simulink model "vehicle_dynamics"  (R2015a)
settings: Solver=ode45  StartTime=0.0  StopTime=10.0  RelTol=1e-3
undefined symbols (not defined in the file): h, I_z, J_wfl, J_wfr, J_wrl, J_wrr, l, l_f, l_r, l_w, m
settings Model: Creator=BML  LastModifiedBy=BML

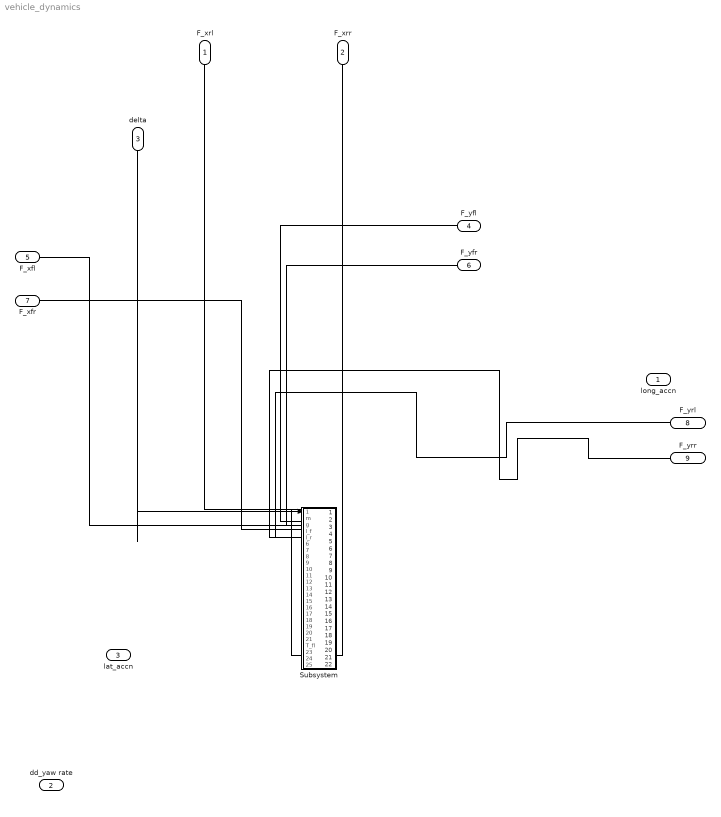
== system vehicle_dynamics ==
  F_xrl : Inport
  F_xrr : Inport  Port=2
  delta : Inport  Port=3
  F_yfl : Inport  Port=4
  F_xfl : Inport  Port=5
  F_yfr : Inport  Port=6
  F_xfr : Inport  Port=7
  F_yrl : Inport  Port=8
  F_yrr : Inport  Port=9
  Subsystem : Subsystem
  long_accn : Outport
  dd_yaw rate : Outport  Port=2
  lat_accn : Outport  Port=3
  wires:
  F_xrl/1 -> ?
  F_xrr/1 -> ?
  delta/1 -> Subsystem/1(delta)
  F_yfl/1 -> ?
  F_xfl/1 -> ?
  F_yfr/1 -> ?
  F_xfr/1 -> ?
  F_yrl/1 -> ?
  F_yrr/1 -> ?
  ? -> long_accn/1
  ? -> dd_yaw rate/1
  ? -> lat_accn/1

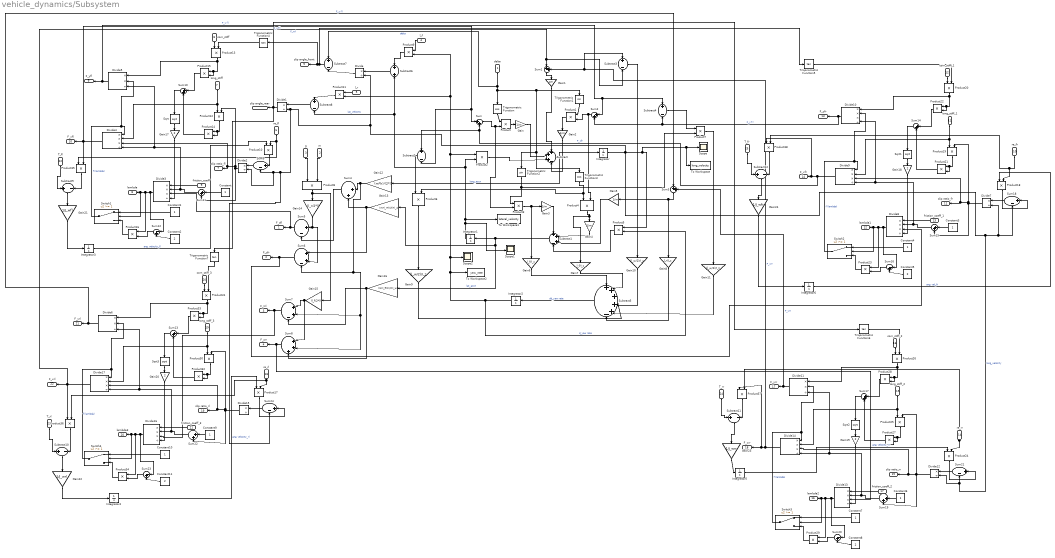
== system vehicle_dynamics/Subsystem ==
  delta : Inport
  m : Inport  Port=2
  g : Inport  Port=3
  l_f : Inport  Port=4
  l_r : Inport  Port=5
  "re_fl " : Inport  Port=6
  "Iong_stiff " : Inport  Port=7
  corn_stiff : Inport  Port=8
  friction_coeff : Inport  Port=9
  "re_fr " : Inport  Port=10
  Iong_stiff_1 : Inport  Port=11
  "corn_stiff_1 " : Inport  Port=12
  friction_coeff_1 : Inport  Port=13
  "re_rr " : Inport  Port=14
  Iong_stiff_2 : Inport  Port=15
  corn_stiff_2 : Inport  Port=16
  friction_coeff_2 : Inport  Port=17
  re_rl : Inport  Port=18
  Iong_stiff_3 : Inport  Port=19
  corn_stiff_3 : Inport  Port=20
  "      friction_coeff_3" : Inport  Port=21
  T_fl : Inport  Port=22
  "T_rl " : Inport  Port=23
  "T_rr " : Inport  Port=24
  "T_fr " : Inport  Port=25
  Constant{,1,3..4,6..7,9..10} (8 alike) : Constant
  Constant{2,5,8,11} (4 alike) : Constant  Value=2
  Divide{,1..2,7,12,15} (6 alike) : Product  Inputs=*/
  Divide{3..4,8..10,13..14,16..17} (9 alike) : Product  Inputs=***/
  Divide11 : Product  Inputs=**/
  Divide5 : Product  Inputs=**/
  Divide6 : Product  Inputs=**/
  Gain{,1..5} (6 alike) : Gain  Gain=1/m
  Gain10 : Gain  Gain=(l_w/2)/I_z
  Gain11 : Gain  Gain=(l_w/2)/I_z
  Gain12 : Gain  Gain=(m*h)/(2*l)
  Gain13 : Gain  Gain=(m*l_r*h)/(l*l_w)
  Gain14 : Gain  Gain=(l_r/2*l)
  Gain15 : Gain  Gain=(l_f/2*l)
  Gain16 : Gain  Gain=(m*l_f*h)/(l*l_w)
  Gain{17..20} (4 alike) : Gain  Gain=2
  Gain21 : Gain  Gain=1/J_wfl
  Gain22 : Gain  Gain=1/J_wrl
  Gain23 : Gain  Gain=1/J_wrr
  Gain24 : Gain  Gain=1/J_wfr
  Gain6 : Gain  Gain=l_f/I_z
  Gain7 : Gain  Gain=l_f/I_z
  Gain8 : Gain  Gain=l_r/I_z
  Gain9 : Gain  Gain=(l_w/2)/I_z
  Integrator{,1..6} (7 alike) : Integrator
  Product{,1..38} (39 alike) : Product
  Scope : Scope
  Scope1 : Scope
  Scope2 : Scope
      settings: SaveName=ScopeData2
  Sqrt{,1..3} (4 alike) : Sqrt  SaturateOnIntegerOverflow=on
  Subtract : Sum  Inputs=+++-
  Subtract1 : Sum  Inputs=+++-
  Subtract{2..4,7..12} (9 alike) : Sum  Inputs=+-
  Subtract5 : Sum  Inputs=+++++-
  Subtract6 : Sum
  Sum{,1..4,10..11,13..15,17,19,22} (13 alike) : Sum  Inputs=|++
  Sum{12,16,20,23} (4 alike) : Sum  Inputs=|-+
  Sum{5,9,18,21,24} (5 alike) : Sum  Inputs=|+-
  Sum6 : Sum  Inputs=|++-
  Sum7 : Sum  Inputs=|++-
  Sum8 : Sum  Inputs=|+++
  Switch{1..4} (4 alike) : Switch  Threshold=1
  To Workspace : ToWorkspace  VariableName=long_velocity  SaveFormat=Timeseries  SampleTime=-1
  To Workspace1 : ToWorkspace  VariableName=lateral_velocity  SaveFormat=Timeseries  SampleTime=-1
  To Workspace2 : ToWorkspace  VariableName=yaw_rate  SaveFormat=Timeseries  SampleTime=-1
  Trigonometric Function : Trigonometry  Operator=cos
  Trigonometric Function1 : Trigonometry
  Trigonometric Function2 : Trigonometry
  Trigonometric Function3 : Trigonometry  Operator=cos
  Trigonometric Function{4..7} (4 alike) : Trigonometry  Operator=tan
  F_zfl : Outport
  F_zfr : Outport  Port=2
  F_zrl : Outport  Port=3
  F_zrr : Outport  Port=4
  slip angle_front : Outport  Port=5
  slip angle_rear : Outport  Port=6
  slip ratio_fl : Outport  Port=7
  lambda : Outport  Port=8
  "F_yfl " : Outport  Port=9
  "F_xfl " : Outport  Port=10
  slip ratio_fr : Outport  Port=11
  lambda1 : Outport  Port=12
  F_yfr : Outport  Port=13
  F_xfr : Outport  Port=14
  slip ratio_rr : Outport  Port=15
  lambda2 : Outport  Port=16
  F_yrr : Outport  Port=17
  F_xrr : Outport  Port=18
  slip ratio_rl : Outport  Port=19
  lambda3 : Outport  Port=20
  F_yrl : Outport  Port=21
  "F_xrl " : Outport  Port=22
  wires:
  Gain10/1 -> Subtract5/4
  Product2/1 -> Subtract/3
  Gain11/1 -> Subtract5/5
  Sum3/1 -> Gain5/1, Gain8/1
  Integrator1/1 -> Scope1/1, Subtract8/2, Subtract6/2, Product2/2, To Workspace1/1  "lat_velocity"
  Subtract3/1 -> Gain10/1
  Gain3/1 -> Subtract1/1
  Product5/1 -> Subtract1/4
  Integrator2/1 -> Product5/2, To Workspace2/1, Scope2/1, Product9/2, Product11/2, Product2/1  "d_yaw rate"
  Trigonometric Function3/1 -> Product6/2, Product4/1
  Product7/1 -> Gain11/1
  Product4/1 -> Gain7/1, Gain4/1
  Trigonometric Function1/1 -> Product1/1
  Gain4/1 -> Subtract1/2
  Product3/1 -> Gain6/1, Gain3/1
  Subtract4/1 -> Product7/1
  Gain/1 -> Subtract/2
  Trigonometric Function/1 -> Product/1
  Sum/1 -> Product3/2, Product/2
  Product/1 -> Gain/1
  Subtract/1 -> Integrator/1, Gain12/1  "long_accn"
  Gain6/1 -> Subtract5/1
  Gain5/1 -> Subtract1/3
  Sum1/1 -> Gain1/1
  Subtract1/1 -> Integrator1/1, Gain13/1, Gain16/1  "lat_accn"
  Gain2/1 -> Subtract/4
  Product1/1 -> Gain2/1
  Trigonometric Function2/1 -> Product3/1, Product7/2
  Sum2/1 -> Product1/2, Product4/2
  Gain8/1 -> Subtract5/6
  Gain7/1 -> Subtract5/2
  Product6/1 -> Gain9/1
  Gain9/1 -> Subtract5/3
  Subtract5/1 -> Integrator2/1  "dd_yaw rate"
  Gain1/1 -> Subtract/1
  Subtract2/1 -> Product6/1
  Gain13/1 -> Sum4/2, Sum6/1
  g/1 -> Product8/1
  m/1 -> Product8/2
  Sum5/1 -> Divide3/3, F_zfl/1
  Gain14/1 -> Sum6/2, Sum5/1
  Product8/1 -> Gain15/1, Gain14/1
  Gain12/1 -> Sum8/2, Sum7/2, Sum6/3, Sum4/1
  Gain15/1 -> Sum8/1, Sum7/1
  Sum4/1 -> Sum5/2
  Gain16/1 -> Sum8/3, Sum7/3
  l_f/1 -> Product9/1
  Product9/1 -> Subtract6/1
  Subtract6/1 -> Divide/1
  delta/1 -> Subtract7/1, Trigonometric Function/1, Trigonometric Function3/1, Trigonometric Function2/1, Trigonometric Function1/1  "delta"
  l_r/1 -> Product11/1
  Product11/1 -> Subtract8/1
  Divide/1 -> Subtract7/2
  Subtract8/1 -> Divide1/1
  Product10/1 -> Sum9/1
  Sum9/1 -> Divide2/1
  "Iong_stiff "/1 -> Divide4/2, Product12/1
  Divide2/1 -> Product12/2, Divide4/3, slip ratio_fl/1, Sum11/2
  corn_stiff/1 -> Product13/1
  Subtract7/1 -> Trigonometric Function5/1, Trigonometric Function4/1, slip angle_front/1
  Product12/1 -> Product14/2, Product14/1
  Trigonometric Function4/1 -> Product13/2
  Product13/1 -> Product15/2, Product15/1, Divide5/1
  Product14/1 -> Sum10/2
  Product15/1 -> Sum10/1
  Sum10/1 -> Sqrt/1
  Sqrt/1 -> Gain17/1
  Constant/1 -> Sum11/1
  Gain17/1 -> Divide3/4
  friction_coeff/1 -> Divide3/1
  Sum11/1 -> Divide5/3, Divide4/4, Divide3/2
  Divide3/1 -> Product16/1, Switch1/2, lambda/1, Sum12/1
  Constant1/1 -> Switch1/1
  Constant2/1 -> Sum12/2
  Sum12/1 -> Product16/2
  Product16/1 -> Switch1/3
  Switch1/1 -> Divide5/2, Divide4/1  "f (lambda)"
  Divide4/1 -> Sum/1, Subtract2/2, "F_xfl "/1, Product35/2  "F_x f l"
  Integrator/1 -> Divide7/2, Sum18/2, Divide12/2, Sum21/2, Sum24/2, Divide2/2, Sum9/2, Divide1/2, Divide/2, To Workspace/1, Scope/1, Product5/1  "long_velocity"
  Product18/1 -> Sum18/1
  Sum18/1 -> Divide7/1
  Iong_stiff_1/1 -> Divide9/2, Product19/1
  Divide7/1 -> Product19/2, Divide9/3, slip ratio_fr/1, Sum15/2
  "corn_stiff_1 "/1 -> Product20/1
  Product19/1 -> Product21/2, Product21/1
  Product20/1 -> Product22/2, Product22/1, Divide10/1
  Product21/1 -> Sum14/2
  Product22/1 -> Sum14/1
  Sum14/1 -> Sqrt1/1
  Sqrt1/1 -> Gain18/1
  Constant3/1 -> Sum15/1
  Gain18/1 -> Divide8/4
  friction_coeff_1/1 -> Divide8/1
  Sum15/1 -> Divide10/4, Divide9/4, Divide8/2
  Divide8/1 -> Product23/1, Switch2/2, lambda1/1, Sum16/1
  Constant4/1 -> Switch2/1
  Constant5/1 -> Sum16/2
  Sum16/1 -> Product23/2
  Product23/1 -> Switch2/3
  Switch2/1 -> Divide10/2, Divide9/1  "f (lambda)"
  Divide9/1 -> Subtract2/1, Sum/2, Product38/1, F_xfr/1  "F_xfr"
  Sum6/1 -> Divide8/3, F_zfr/1
  Trigonometric Function5/1 -> Product20/2
  Product24/1 -> Sum21/1
  Sum21/1 -> Divide12/1
  Iong_stiff_2/1 -> Divide14/2, Product25/1
  Divide12/1 -> Product25/2, Divide14/3, slip ratio_rr/1, Sum19/2
  corn_stiff_2/1 -> Product26/1
  Product25/1 -> Product27/2, Product27/1
  Product26/1 -> Product28/2, Product28/1, Divide11/1
  Product27/1 -> Sum17/2
  Product28/1 -> Sum17/1
  Sum17/1 -> Sqrt2/1
  Sqrt2/1 -> Gain19/1
  Constant6/1 -> Sum19/1
  Gain19/1 -> Divide13/4
  friction_coeff_2/1 -> Divide13/1
  Sum19/1 -> Divide11/3, Divide14/4, Divide13/2
  Divide13/1 -> Product29/1, Switch3/2, lambda2/1, Sum20/1
  Constant7/1 -> Switch3/1
  Constant8/1 -> Sum20/2
  Sum20/1 -> Product29/2
  Product29/1 -> Switch3/3
  Switch3/1 -> Divide11/2, Divide14/1  "f (lambda)"
  Divide11/1 -> Sum3/2, F_yrr/1  "F_yrr"
  Trigonometric Function6/1 -> Product26/2
  Sum8/1 -> Divide13/3, F_zrr/1
  re_rl/1 -> Product36/2, Product17/2
  Product17/1 -> Sum24/1
  Sum24/1 -> Divide15/1
  Iong_stiff_3/1 -> Divide17/2, Product30/1
  Divide15/1 -> Product30/2, Divide17/3, slip ratio_rl/1, Sum22/2
  corn_stiff_3/1 -> Product31/1
  Product30/1 -> Product32/2, Product32/1
  Product31/1 -> Product33/2, Product33/1, Divide6/1
  Product32/1 -> Sum13/2
  Product33/1 -> Sum13/1
  Sum13/1 -> Sqrt3/1
  Sqrt3/1 -> Gain20/1
  Constant9/1 -> Sum22/1
  Gain20/1 -> Divide16/4
  "      friction_coeff_3"/1 -> Divide16/1
  Sum22/1 -> Divide6/3, Divide17/4, Divide16/2
  Divide16/1 -> Product34/1, Switch4/2, lambda3/1, Sum23/1
  Constant10/1 -> Switch4/1
  Constant11/1 -> Sum23/2
  Sum23/1 -> Product34/2
  Product34/1 -> Switch4/3
  Switch4/1 -> Divide6/2, Divide17/1  "f (lambda)"
  Trigonometric Function7/1 -> Product31/2
  Divide1/1 -> Trigonometric Function7/1, Trigonometric Function6/1, slip angle_rear/1
  Sum7/1 -> Divide16/3, F_zrl/1
  "re_fl "/1 -> Product10/2, Product35/1
  T_fl/1 -> Subtract9/1
  Product35/1 -> Subtract9/2
  Subtract9/1 -> Gain21/1
  Gain21/1 -> Integrator3/1
  Integrator3/1 -> Product10/1  "ang. velocity_fl"
  Subtract10/1 -> Gain22/1
  "T_rl "/1 -> Subtract10/1
  Product36/1 -> Subtract10/2
  Gain22/1 -> Integrator4/1
  Integrator4/1 -> Product17/1  "ang. velocity_rl"
  Subtract11/1 -> Gain23/1
  "T_rr "/1 -> Subtract11/1
  Product37/1 -> Subtract11/2
  "re_rr "/1 -> Product24/2, Product37/2
  Gain23/1 -> Integrator5/1
  Integrator5/1 -> Product24/1  "ang. velocity_rr"
  Subtract12/1 -> Gain24/1
  Product38/1 -> Subtract12/2
  "re_fr "/1 -> Product18/2, Product38/2
  "T_fr "/1 -> Subtract12/1
  Gain24/1 -> Integrator6/1
  Integrator6/1 -> Product18/1  "ang. vel_fr"
  Divide14/1 -> Sum1/2, Subtract3/1, F_xrr/1, Product37/1  "F_xrr"
  Divide17/1 -> "F_xrl "/1, Subtract3/2, Sum1/1, Product36/1  "F_xrl"
  Divide10/1 -> Sum2/2, Subtract4/2, F_yfr/1  "F_y f r"
  Divide5/1 -> Sum2/1, Subtract4/1, "F_yfl "/1  "F_y f l"
  Divide6/1 -> Sum3/1, F_yrl/1  "F_y f l"
